simulink model "hw1"  (R2020b)
settings: Solver=VariableStepAuto  StartTime=0.0  StopTime=0.4  RelTol=1e-3
values from neighbouring files (symbols this model uses):
  J = 3.35e-6    (= 3.35e-06)    [params.m]
  Kphi = 25.9e-3    (= 0.0259)    [params.m]
  Kv = 4.63e-6    (= 4.63e-06)    [params.m]
  La = 0.119e-3    (= 0.000119)    [params.m]
  Ra = 0.611    [params.m]
settings Model: Creator=Balazs  LastModifiedBy=Balazs

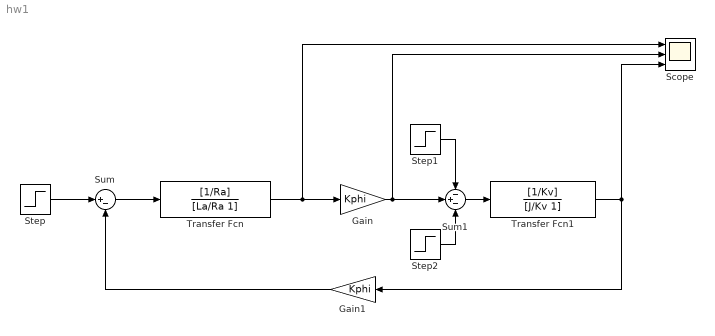
== system hw1 ==
  Gain : Gain  Gain=Kphi
  Gain1 : Gain  Gain=Kphi
  Scope : Scope  NumInputPorts=3
  Step : Step  Time=0.1  After=24  SampleTime=0
  Step1 : Step  Time=0.2  After=0.028  SampleTime=0
  Step2 : Step  Time=0.3  After=0.028  SampleTime=0
  Sum : Sum  Inputs=|+-
  Sum1 : Sum  Inputs=-+-
  Transfer Fcn : TransferFcn  Numerator=[1/Ra]  Denominator=[La/Ra 1]
  Transfer Fcn1 : TransferFcn  Numerator=[1/Kv]  Denominator=[J/Kv 1]
  wires:
  Sum/1 -> Transfer Fcn/1
  Transfer Fcn/1 -> Scope/1, Gain/1
  Gain/1 -> Scope/2, Sum1/2
  Sum1/1 -> Transfer Fcn1/1
  Transfer Fcn1/1 -> Gain1/1, Scope/3
  Gain1/1 -> Sum/2
  Step1/1 -> Sum1/1
  Step/1 -> Sum/1
  Step2/1 -> Sum1/3
